simulink model "c00005M_harness"  (R2018a)
settings: Solver=ode3  StartTime=0.0  StopTime=10.0  RelTol=1e-3  EnableMultiTasking=on
undefined symbols (not defined in the file): b, DiscIntNeverNeededParam, J, K, L, PosMinimaW3, PosMinimaW4, R, sigbuilder_block
(part 19 of 75)

== system c00005M_harness/M080/Cyber ==
  note: Sensors
  note: Inputs For Window1
  note: Inputs for Window 2
  note: Inputs for window 3
  note: Inputs for window 4
  note: Users
  note: Users
  note: Sensors
  note: Users
  note: Sensors
  note: Users
  note: Sensors
  note: USERS
      | ---------------------------------
      | 0: None
      | 1: Ventana Arriba
      | 2: Ventana hasta arriba
      | 3: Ventana abajo
      | 4: Ventana hasta abajo
  note: 1: SUBE
      | 0: PARADO
      | -1 BAJA
  note: D = Driver (W1)
      | P1 = Passenger 1 (W2)
      | P2 = Passenger 2 (W3)
      | P3 = Passenger 3 (W4)
      | O = Obstacle
      | C = Control
      | Pri = Prioritizer
      | LD = LockDriver
      | PosW = PositionWindow
      | WL = WindowLogic
      | OW = ObstacleWindow
      | CWXC = ControlWindowXCentralized
      | S = Sensor
      | L = Lock
      | WPos = WindowPosition
      | M = Memory
      | InW = InputWindow
      | WIn = WindowInput
  PosW1 : Inport
  PosW2 : Inport  Port=2
  PosW3 : Inport  Port=3
  PosW4 : Inport  Port=4
  DW1 : Inport  Port=5
  DW3 : Inport  Port=6
  DW4 : Inport  Port=7
  P1W2 : Inport  Port=8
  P2W3 : Inport  Port=9
  P1W3 : Inport  Port=10
  P3W4 : Inport  Port=11
  OW1 : Inport  Port=12
  OW2 : Inport  Port=13
  OW3 : Inport  Port=14
  OW4 : Inport  Port=15
  LD : Inport  Port=16
  CW1C : Inport  Port=17
  CW2C : Inport  Port=18
  CW3C : Inport  Port=19
  CW4C : Inport  Port=20
  Pri : Subsystem
  Pri1 : Subsystem
  Pri3 : Subsystem
  Pri4 : Subsystem
  WL : Subsystem
  WL1 : Subsystem
  WL2 : Subsystem
  WL3 : Subsystem
  W1 : Outport
  W2 : Outport  Port=2
  W3 : Outport  Port=3
  W4 : Outport  Port=4
  wires:
  CW4C/1 -> Pri4/3(CW4C)
  CW3C/1 -> Pri1/4(CW3C)
  CW2C/1 -> Pri/2(CW2C)
  CW1C/1 -> Pri3/2(CW1C)
  Pri3/1(User) -> WL/2(User)
  WL3/1(WindowLogicOutput) -> W4/1
  WL2/1(WindowLogicOutput) -> W3/1
  Pri4/1(User) -> WL3/2(User)
  OW4/1 -> WL3/3(OW)
  PosW4/1 -> WL3/1(WPos)
  P3W4/1 -> Pri4/2(P)
  DW4/1 -> Pri4/1(D)
  P1W3/1 -> Pri1/3(P1)
  P2W3/1 -> Pri1/2(P)
  DW3/1 -> Pri1/1(D)
  OW3/1 -> WL2/3(OW)
  PosW3/1 -> WL2/1(WPos)
  Pri1/1(User) -> WL2/2(User)
  WL1/1(WindowLogicOutput) -> W2/1
  OW2/1 -> WL1/3(OW)
  PosW2/1 -> WL1/1(WPos)
  P1W2/1 -> Pri/1(P)
  Pri/1(User) -> WL1/2(User)
  WL/1(WindowLogicOutput) -> W1/1
  DW1/1 -> Pri3/1(D)
  OW1/1 -> WL/3(OW)
  PosW1/1 -> WL/1(WPos)
  LD/1 -> WL3/4(L)

== system c00005M_harness/M080/Physical ==
  InW1 : Inport
  InW2 : Inport  Port=2
  InW3 : Inport  Port=3
  InW4 : Inport  Port=4
  W : Subsystem
  W5 : Subsystem
  W6 : Subsystem
  W7 : Subsystem
  W1 : Outport
  W2 : Outport  Port=2
  W3 : Outport  Port=3
  W4 : Outport  Port=4
  wires:
  W7/1(WPos) -> W4/1
  W6/1(WPos) -> W3/1
  W5/1(WPos) -> W2/1
  W/1(WPos) -> W1/1
  InW4/1 -> W7/1(WIn)
  InW3/1 -> W6/1(WIn)
  InW2/1 -> W5/1(WIn)
  InW1/1 -> W/1(WIn)

== system c00005M_harness/M080/S1 ==
  PhyMeasure : Inport
  SensorOut : Outport
  wires:
  PhyMeasure/1 -> SensorOut/1

== system c00005M_harness/M080/S2 ==
  PhyMeasure : Inport
  SensorOut : Outport
  wires:
  PhyMeasure/1 -> SensorOut/1

== system c00005M_harness/M080/S3 ==
  PhyMeasure : Inport
  SensorOut : Outport
  wires:
  PhyMeasure/1 -> SensorOut/1

== system c00005M_harness/M080/S4 ==
  PhyMeasure : Inport
  SensorOut : Outport
  wires:
  PhyMeasure/1 -> SensorOut/1

== system c00005M_harness/M081/Cyber ==
  note: Sensors
  note: Inputs For Window1
  note: Inputs for Window 2
  note: Inputs for window 3
  note: Inputs for window 4
  note: Users
  note: Users
  note: Sensors
  note: Users
  note: Sensors
  note: Users
  note: Sensors
  note: USERS
      | ---------------------------------
      | 0: None
      | 1: Ventana Arriba
      | 2: Ventana hasta arriba
      | 3: Ventana abajo
      | 4: Ventana hasta abajo
  note: 1: SUBE
      | 0: PARADO
      | -1 BAJA
  note: D = Driver (W1)
      | P1 = Passenger 1 (W2)
      | P2 = Passenger 2 (W3)
      | P3 = Passenger 3 (W4)
      | O = Obstacle
      | C = Control
      | Pri = Prioritizer
      | LD = LockDriver
      | PosW = PositionWindow
      | WL = WindowLogic
      | OW = ObstacleWindow
      | CWXC = ControlWindowXCentralized
      | S = Sensor
      | L = Lock
      | WPos = WindowPosition
      | M = Memory
      | InW = InputWindow
      | WIn = WindowInput
  PosW1 : Inport
  PosW2 : Inport  Port=2
  PosW3 : Inport  Port=3
  PosW4 : Inport  Port=4
  DW1 : Inport  Port=5
  DW3 : Inport  Port=6
  DW4 : Inport  Port=7
  P1W2 : Inport  Port=8
  P2W3 : Inport  Port=9
  P1W3 : Inport  Port=10
  P3W4 : Inport  Port=11
  OW1 : Inport  Port=12
  OW2 : Inport  Port=13
  OW3 : Inport  Port=14
  OW4 : Inport  Port=15
  LD : Inport  Port=16
  CW1C : Inport  Port=17
  CW2C : Inport  Port=18
  CW3C : Inport  Port=19
  CW4C : Inport  Port=20
  Pri : Subsystem
  Pri1 : Subsystem
  Pri3 : Subsystem
  Pri4 : Subsystem
  WL : Subsystem
  WL1 : Subsystem
  WL2 : Subsystem
  WL3 : Subsystem
  W1 : Outport
  W2 : Outport  Port=2
  W3 : Outport  Port=3
  W4 : Outport  Port=4
  wires:
  CW4C/1 -> Pri4/3(CW4C)
  CW3C/1 -> Pri1/4(CW3C)
  CW2C/1 -> Pri/2(CW2C)
  CW1C/1 -> Pri3/2(CW1C)
  Pri3/1(User) -> WL/2(User)
  WL3/1(WindowLogicOutput) -> W4/1
  WL2/1(WindowLogicOutput) -> W3/1
  Pri4/1(User) -> WL3/2(User)
  OW4/1 -> WL3/3(OW)
  PosW4/1 -> WL3/1(WPos)
  P3W4/1 -> Pri4/2(P)
  DW4/1 -> Pri4/1(D)
  P1W3/1 -> Pri1/3(P1)
  P2W3/1 -> Pri1/2(P)
  DW3/1 -> Pri1/1(D)
  OW3/1 -> WL2/3(OW)
  PosW3/1 -> WL2/1(WPos)
  Pri1/1(User) -> WL2/2(User)
  WL1/1(WindowLogicOutput) -> W2/1
  OW2/1 -> WL1/3(OW)
  PosW2/1 -> WL1/1(WPos)
  P1W2/1 -> Pri/1(P)
  Pri/1(User) -> WL1/2(User)
  WL/1(WindowLogicOutput) -> W1/1
  DW1/1 -> Pri3/1(D)
  OW1/1 -> WL/3(OW)
  PosW1/1 -> WL/1(WPos)
  LD/1 -> WL3/4(L)

== system c00005M_harness/M081/Physical ==
  InW1 : Inport
  InW2 : Inport  Port=2
  InW3 : Inport  Port=3
  InW4 : Inport  Port=4
  W : Subsystem
  W5 : Subsystem
  W6 : Subsystem
  W7 : Subsystem
  W1 : Outport
  W2 : Outport  Port=2
  W3 : Outport  Port=3
  W4 : Outport  Port=4
  wires:
  W7/1(WPos) -> W4/1
  W6/1(WPos) -> W3/1
  W5/1(WPos) -> W2/1
  W/1(WPos) -> W1/1
  InW4/1 -> W7/1(WIn)
  InW3/1 -> W6/1(WIn)
  InW2/1 -> W5/1(WIn)
  InW1/1 -> W/1(WIn)

== system c00005M_harness/M081/S1 ==
  PhyMeasure : Inport
  SensorOut : Outport
  wires:
  PhyMeasure/1 -> SensorOut/1

== system c00005M_harness/M081/S2 ==
  PhyMeasure : Inport
  SensorOut : Outport
  wires:
  PhyMeasure/1 -> SensorOut/1

== system c00005M_harness/M081/S3 ==
  PhyMeasure : Inport
  SensorOut : Outport
  wires:
  PhyMeasure/1 -> SensorOut/1

== system c00005M_harness/M081/S4 ==
  PhyMeasure : Inport
  SensorOut : Outport
  wires:
  PhyMeasure/1 -> SensorOut/1

== system c00005M_harness/M082/Cyber ==
  note: Sensors
  note: Inputs For Window1
  note: Inputs for Window 2
  note: Inputs for window 3
  note: Inputs for window 4
  note: Users
  note: Users
  note: Sensors
  note: Users
  note: Sensors
  note: Users
  note: Sensors
  note: USERS
      | ---------------------------------
      | 0: None
      | 1: Ventana Arriba
      | 2: Ventana hasta arriba
      | 3: Ventana abajo
      | 4: Ventana hasta abajo
  note: 1: SUBE
      | 0: PARADO
      | -1 BAJA
  note: D = Driver (W1)
      | P1 = Passenger 1 (W2)
      | P2 = Passenger 2 (W3)
      | P3 = Passenger 3 (W4)
      | O = Obstacle
      | C = Control
      | Pri = Prioritizer
      | LD = LockDriver
      | PosW = PositionWindow
      | WL = WindowLogic
      | OW = ObstacleWindow
      | CWXC = ControlWindowXCentralized
      | S = Sensor
      | L = Lock
      | WPos = WindowPosition
      | M = Memory
      | InW = InputWindow
      | WIn = WindowInput
  PosW1 : Inport
  PosW2 : Inport  Port=2
  PosW3 : Inport  Port=3
  PosW4 : Inport  Port=4
  DW1 : Inport  Port=5
  DW3 : Inport  Port=6
  DW4 : Inport  Port=7
  P1W2 : Inport  Port=8
  P2W3 : Inport  Port=9
  P1W3 : Inport  Port=10
  P3W4 : Inport  Port=11
  OW1 : Inport  Port=12
  OW2 : Inport  Port=13
  OW3 : Inport  Port=14
  OW4 : Inport  Port=15
  LD : Inport  Port=16
  CW1C : Inport  Port=17
  CW2C : Inport  Port=18
  CW3C : Inport  Port=19
  CW4C : Inport  Port=20
  Pri : Subsystem
  Pri1 : Subsystem
  Pri3 : Subsystem
  Pri4 : Subsystem
  WL : Subsystem
  WL1 : Subsystem
  WL2 : Subsystem
  WL3 : Subsystem
  W1 : Outport
  W2 : Outport  Port=2
  W3 : Outport  Port=3
  W4 : Outport  Port=4
  wires:
  CW4C/1 -> Pri4/3(CW4C)
  CW3C/1 -> Pri1/4(CW3C)
  CW2C/1 -> Pri/2(CW2C)
  CW1C/1 -> Pri3/2(CW1C)
  Pri3/1(User) -> WL/2(User)
  WL3/1(WindowLogicOutput) -> W4/1
  WL2/1(WindowLogicOutput) -> W3/1
  Pri4/1(User) -> WL3/2(User)
  OW4/1 -> WL3/3(OW)
  PosW4/1 -> WL3/1(WPos)
  P3W4/1 -> Pri4/2(P)
  DW4/1 -> Pri4/1(D)
  P1W3/1 -> Pri1/3(P1)
  P2W3/1 -> Pri1/2(P)
  DW3/1 -> Pri1/1(D)
  OW3/1 -> WL2/3(OW)
  PosW3/1 -> WL2/1(WPos)
  Pri1/1(User) -> WL2/2(User)
  WL1/1(WindowLogicOutput) -> W2/1
  OW2/1 -> WL1/3(OW)
  PosW2/1 -> WL1/1(WPos)
  P1W2/1 -> Pri/1(P)
  Pri/1(User) -> WL1/2(User)
  WL/1(WindowLogicOutput) -> W1/1
  DW1/1 -> Pri3/1(D)
  OW1/1 -> WL/3(OW)
  PosW1/1 -> WL/1(WPos)
  LD/1 -> WL3/4(L)

== system c00005M_harness/M082/Physical ==
  InW1 : Inport
  InW2 : Inport  Port=2
  InW3 : Inport  Port=3
  InW4 : Inport  Port=4
  W : Subsystem
  W5 : Subsystem
  W6 : Subsystem
  W7 : Subsystem
  W1 : Outport
  W2 : Outport  Port=2
  W3 : Outport  Port=3
  W4 : Outport  Port=4
  wires:
  W7/1(WPos) -> W4/1
  W6/1(WPos) -> W3/1
  W5/1(WPos) -> W2/1
  W/1(WPos) -> W1/1
  InW4/1 -> W7/1(WIn)
  InW3/1 -> W6/1(WIn)
  InW2/1 -> W5/1(WIn)
  InW1/1 -> W/1(WIn)

== system c00005M_harness/M082/S1 ==
  PhyMeasure : Inport
  SensorOut : Outport
  wires:
  PhyMeasure/1 -> SensorOut/1

== system c00005M_harness/M082/S2 ==
  PhyMeasure : Inport
  SensorOut : Outport
  wires:
  PhyMeasure/1 -> SensorOut/1

== system c00005M_harness/M082/S3 ==
  PhyMeasure : Inport
  SensorOut : Outport
  wires:
  PhyMeasure/1 -> SensorOut/1

== system c00005M_harness/M082/S4 ==
  PhyMeasure : Inport
  SensorOut : Outport
  wires:
  PhyMeasure/1 -> SensorOut/1

== system c00005M_harness/M083/Cyber ==
  note: Sensors
  note: Inputs For Window1
  note: Inputs for Window 2
  note: Inputs for window 3
  note: Inputs for window 4
  note: Users
  note: Users
  note: Sensors
  note: Users
  note: Sensors
  note: Users
  note: Sensors
  note: USERS
      | ---------------------------------
      | 0: None
      | 1: Ventana Arriba
      | 2: Ventana hasta arriba
      | 3: Ventana abajo
      | 4: Ventana hasta abajo
  note: 1: SUBE
      | 0: PARADO
      | -1 BAJA
  note: D = Driver (W1)
      | P1 = Passenger 1 (W2)
      | P2 = Passenger 2 (W3)
      | P3 = Passenger 3 (W4)
      | O = Obstacle
      | C = Control
      | Pri = Prioritizer
      | LD = LockDriver
      | PosW = PositionWindow
      | WL = WindowLogic
      | OW = ObstacleWindow
      | CWXC = ControlWindowXCentralized
      | S = Sensor
      | L = Lock
      | WPos = WindowPosition
      | M = Memory
      | InW = InputWindow
      | WIn = WindowInput
  PosW1 : Inport
  PosW2 : Inport  Port=2
  PosW3 : Inport  Port=3
  PosW4 : Inport  Port=4
  DW1 : Inport  Port=5
  DW3 : Inport  Port=6
  DW4 : Inport  Port=7
  P1W2 : Inport  Port=8
  P2W3 : Inport  Port=9
  P1W3 : Inport  Port=10
  P3W4 : Inport  Port=11
  OW1 : Inport  Port=12
  OW2 : Inport  Port=13
  OW3 : Inport  Port=14
  OW4 : Inport  Port=15
  LD : Inport  Port=16
  CW1C : Inport  Port=17
  CW2C : Inport  Port=18
  CW3C : Inport  Port=19
  CW4C : Inport  Port=20
  Pri : Subsystem
  Pri1 : Subsystem
  Pri3 : Subsystem
  Pri4 : Subsystem
  WL : Subsystem
  WL1 : Subsystem
  WL2 : Subsystem
  WL3 : Subsystem
  W1 : Outport
  W2 : Outport  Port=2
  W3 : Outport  Port=3
  W4 : Outport  Port=4
  wires:
  CW4C/1 -> Pri4/3(CW4C)
  CW3C/1 -> Pri1/4(CW3C)
  CW2C/1 -> Pri/2(CW2C)
  CW1C/1 -> Pri3/2(CW1C)
  Pri3/1(User) -> WL/2(User)
  WL3/1(WindowLogicOutput) -> W4/1
  WL2/1(WindowLogicOutput) -> W3/1
  Pri4/1(User) -> WL3/2(User)
  OW4/1 -> WL3/3(OW)
  PosW4/1 -> WL3/1(WPos)
  P3W4/1 -> Pri4/2(P)
  DW4/1 -> Pri4/1(D)
  P1W3/1 -> Pri1/3(P1)
  P2W3/1 -> Pri1/2(P)
  DW3/1 -> Pri1/1(D)
  OW3/1 -> WL2/3(OW)
  PosW3/1 -> WL2/1(WPos)
  Pri1/1(User) -> WL2/2(User)
  WL1/1(WindowLogicOutput) -> W2/1
  OW2/1 -> WL1/3(OW)
  PosW2/1 -> WL1/1(WPos)
  P1W2/1 -> Pri/1(P)
  Pri/1(User) -> WL1/2(User)
  WL/1(WindowLogicOutput) -> W1/1
  DW1/1 -> Pri3/1(D)
  OW1/1 -> WL/3(OW)
  PosW1/1 -> WL/1(WPos)
  LD/1 -> WL3/4(L)

== system c00005M_harness/M083/Physical ==
  InW1 : Inport
  InW2 : Inport  Port=2
  InW3 : Inport  Port=3
  InW4 : Inport  Port=4
  W : Subsystem
  W5 : Subsystem
  W6 : Subsystem
  W7 : Subsystem
  W1 : Outport
  W2 : Outport  Port=2
  W3 : Outport  Port=3
  W4 : Outport  Port=4
  wires:
  W7/1(WPos) -> W4/1
  W6/1(WPos) -> W3/1
  W5/1(WPos) -> W2/1
  W/1(WPos) -> W1/1
  InW4/1 -> W7/1(WIn)
  InW3/1 -> W6/1(WIn)
  InW2/1 -> W5/1(WIn)
  InW1/1 -> W/1(WIn)

== system c00005M_harness/M083/S1 ==
  PhyMeasure : Inport
  SensorOut : Outport
  wires:
  PhyMeasure/1 -> SensorOut/1

== system c00005M_harness/M083/S2 ==
  PhyMeasure : Inport
  SensorOut : Outport
  wires:
  PhyMeasure/1 -> SensorOut/1

== system c00005M_harness/M083/S3 ==
  PhyMeasure : Inport
  SensorOut : Outport
  wires:
  PhyMeasure/1 -> SensorOut/1

== system c00005M_harness/M083/S4 ==
  PhyMeasure : Inport
  SensorOut : Outport
  wires:
  PhyMeasure/1 -> SensorOut/1

== system c00005M_harness/M084/Cyber ==
  note: Sensors
  note: Inputs For Window1
  note: Inputs for Window 2
  note: Inputs for window 3
  note: Inputs for window 4
  note: Users
  note: Users
  note: Sensors
  note: Users
  note: Sensors
  note: Users
  note: Sensors
  note: USERS
      | ---------------------------------
      | 0: None
      | 1: Ventana Arriba
      | 2: Ventana hasta arriba
      | 3: Ventana abajo
      | 4: Ventana hasta abajo
  note: 1: SUBE
      | 0: PARADO
      | -1 BAJA
  note: D = Driver (W1)
      | P1 = Passenger 1 (W2)
      | P2 = Passenger 2 (W3)
      | P3 = Passenger 3 (W4)
      | O = Obstacle
      | C = Control
      | Pri = Prioritizer
      | LD = LockDriver
      | PosW = PositionWindow
      | WL = WindowLogic
      | OW = ObstacleWindow
      | CWXC = ControlWindowXCentralized
      | S = Sensor
      | L = Lock
      | WPos = WindowPosition
      | M = Memory
      | InW = InputWindow
      | WIn = WindowInput
  PosW1 : Inport
  PosW2 : Inport  Port=2
  PosW3 : Inport  Port=3
  PosW4 : Inport  Port=4
  DW1 : Inport  Port=5
  DW3 : Inport  Port=6
  DW4 : Inport  Port=7
  P1W2 : Inport  Port=8
  P2W3 : Inport  Port=9
  P1W3 : Inport  Port=10
  P3W4 : Inport  Port=11
  OW1 : Inport  Port=12
  OW2 : Inport  Port=13
  OW3 : Inport  Port=14
  OW4 : Inport  Port=15
  LD : Inport  Port=16
  CW1C : Inport  Port=17
  CW2C : Inport  Port=18
  CW3C : Inport  Port=19
  CW4C : Inport  Port=20
  Pri : Subsystem
  Pri1 : Subsystem
  Pri3 : Subsystem
  Pri4 : Subsystem
  WL : Subsystem
  WL1 : Subsystem
  WL2 : Subsystem
  WL3 : Subsystem
  W1 : Outport
  W2 : Outport  Port=2
  W3 : Outport  Port=3
  W4 : Outport  Port=4
  wires:
  CW4C/1 -> Pri4/3(CW4C)
  CW3C/1 -> Pri1/4(CW3C)
  CW2C/1 -> Pri/2(CW2C)
  CW1C/1 -> Pri3/2(CW1C)
  Pri3/1(User) -> WL/2(User)
  WL3/1(WindowLogicOutput) -> W4/1
  WL2/1(WindowLogicOutput) -> W3/1
  Pri4/1(User) -> WL3/2(User)
  OW4/1 -> WL3/3(OW)
  PosW4/1 -> WL3/1(WPos)
  P3W4/1 -> Pri4/2(P)
  DW4/1 -> Pri4/1(D)
  P1W3/1 -> Pri1/3(P1)
  P2W3/1 -> Pri1/2(P)
  DW3/1 -> Pri1/1(D)
  OW3/1 -> WL2/3(OW)
  PosW3/1 -> WL2/1(WPos)
  Pri1/1(User) -> WL2/2(User)
  WL1/1(WindowLogicOutput) -> W2/1
  OW2/1 -> WL1/3(OW)
  PosW2/1 -> WL1/1(WPos)
  P1W2/1 -> Pri/1(P)
  Pri/1(User) -> WL1/2(User)
  WL/1(WindowLogicOutput) -> W1/1
  DW1/1 -> Pri3/1(D)
  OW1/1 -> WL/3(OW)
  PosW1/1 -> WL/1(WPos)
  LD/1 -> WL3/4(L)

== system c00005M_harness/M084/Physical ==
  InW1 : Inport
  InW2 : Inport  Port=2
  InW3 : Inport  Port=3
  InW4 : Inport  Port=4
  W : Subsystem
  W5 : Subsystem
  W6 : Subsystem
  W7 : Subsystem
  W1 : Outport
  W2 : Outport  Port=2
  W3 : Outport  Port=3
  W4 : Outport  Port=4
  wires:
  W7/1(WPos) -> W4/1
  W6/1(WPos) -> W3/1
  W5/1(WPos) -> W2/1
  W/1(WPos) -> W1/1
  InW4/1 -> W7/1(WIn)
  InW3/1 -> W6/1(WIn)
  InW2/1 -> W5/1(WIn)
  InW1/1 -> W/1(WIn)

== system c00005M_harness/M084/S1 ==
  PhyMeasure : Inport
  SensorOut : Outport
  wires:
  PhyMeasure/1 -> SensorOut/1

== system c00005M_harness/M084/S2 ==
  PhyMeasure : Inport
  SensorOut : Outport
  wires:
  PhyMeasure/1 -> SensorOut/1

== system c00005M_harness/M084/S3 ==
  PhyMeasure : Inport
  SensorOut : Outport
  wires:
  PhyMeasure/1 -> SensorOut/1

== system c00005M_harness/M084/S4 ==
  PhyMeasure : Inport
  SensorOut : Outport
  wires:
  PhyMeasure/1 -> SensorOut/1

== system c00005M_harness/M085/Cyber ==
  note: Sensors
  note: Inputs For Window1
  note: Inputs for Window 2
  note: Inputs for window 3
  note: Inputs for window 4
  note: Users
  note: Users
  note: Sensors
  note: Users
  note: Sensors
  note: Users
  note: Sensors
  note: USERS
      | ---------------------------------
      | 0: None
      | 1: Ventana Arriba
      | 2: Ventana hasta arriba
      | 3: Ventana abajo
      | 4: Ventana hasta abajo
  note: 1: SUBE
      | 0: PARADO
      | -1 BAJA
  note: D = Driver (W1)
      | P1 = Passenger 1 (W2)
      | P2 = Passenger 2 (W3)
      | P3 = Passenger 3 (W4)
      | O = Obstacle
      | C = Control
      | Pri = Prioritizer
      | LD = LockDriver
      | PosW = PositionWindow
      | WL = WindowLogic
      | OW = ObstacleWindow
      | CWXC = ControlWindowXCentralized
      | S = Sensor
      | L = Lock
      | WPos = WindowPosition
      | M = Memory
      | InW = InputWindow
      | WIn = WindowInput
  PosW1 : Inport
  PosW2 : Inport  Port=2
  PosW3 : Inport  Port=3
  PosW4 : Inport  Port=4
  DW1 : Inport  Port=5
  DW3 : Inport  Port=6
  DW4 : Inport  Port=7
  P1W2 : Inport  Port=8
  P2W3 : Inport  Port=9
  P1W3 : Inport  Port=10
  P3W4 : Inport  Port=11
  OW1 : Inport  Port=12
  OW2 : Inport  Port=13
  OW3 : Inport  Port=14
  OW4 : Inport  Port=15
  LD : Inport  Port=16
  CW1C : Inport  Port=17
  CW2C : Inport  Port=18
  CW3C : Inport  Port=19
  CW4C : Inport  Port=20
  Pri : Subsystem
  Pri1 : Subsystem
  Pri3 : Subsystem
  Pri4 : Subsystem
  WL : Subsystem
  WL1 : Subsystem
  WL2 : Subsystem
  WL3 : Subsystem
  W1 : Outport
  W2 : Outport  Port=2
  W3 : Outport  Port=3
  W4 : Outport  Port=4
  wires:
  CW4C/1 -> Pri4/3(CW4C)
  CW3C/1 -> Pri1/4(CW3C)
  CW2C/1 -> Pri/2(CW2C)
  CW1C/1 -> Pri3/2(CW1C)
  Pri3/1(User) -> WL/2(User)
  WL3/1(WindowLogicOutput) -> W4/1
  WL2/1(WindowLogicOutput) -> W3/1
  Pri4/1(User) -> WL3/2(User)
  OW4/1 -> WL3/3(OW)
  PosW4/1 -> WL3/1(WPos)
  P3W4/1 -> Pri4/2(P)
  DW4/1 -> Pri4/1(D)
  P1W3/1 -> Pri1/3(P1)
  P2W3/1 -> Pri1/2(P)
  DW3/1 -> Pri1/1(D)
  OW3/1 -> WL2/3(OW)
  PosW3/1 -> WL2/1(WPos)
  Pri1/1(User) -> WL2/2(User)
  WL1/1(WindowLogicOutput) -> W2/1
  OW2/1 -> WL1/3(OW)
  PosW2/1 -> WL1/1(WPos)
  P1W2/1 -> Pri/1(P)
  Pri/1(User) -> WL1/2(User)
  WL/1(WindowLogicOutput) -> W1/1
  DW1/1 -> Pri3/1(D)
  OW1/1 -> WL/3(OW)
  PosW1/1 -> WL/1(WPos)
  LD/1 -> WL3/4(L)

== system c00005M_harness/M085/Physical ==
  InW1 : Inport
  InW2 : Inport  Port=2
  InW3 : Inport  Port=3
  InW4 : Inport  Port=4
  W : Subsystem
  W5 : Subsystem
  W6 : Subsystem
  W7 : Subsystem
  W1 : Outport
  W2 : Outport  Port=2
  W3 : Outport  Port=3
  W4 : Outport  Port=4
  wires:
  W7/1(WPos) -> W4/1
  W6/1(WPos) -> W3/1
  W5/1(WPos) -> W2/1
  W/1(WPos) -> W1/1
  InW4/1 -> W7/1(WIn)
  InW3/1 -> W6/1(WIn)
  InW2/1 -> W5/1(WIn)
  InW1/1 -> W/1(WIn)

== system c00005M_harness/M085/S1 ==
  PhyMeasure : Inport
  SensorOut : Outport
  wires:
  PhyMeasure/1 -> SensorOut/1

== system c00005M_harness/M085/S2 ==
  PhyMeasure : Inport
  SensorOut : Outport
  wires:
  PhyMeasure/1 -> SensorOut/1

== system c00005M_harness/M085/S3 ==
  PhyMeasure : Inport
  SensorOut : Outport
  wires:
  PhyMeasure/1 -> SensorOut/1

== system c00005M_harness/M085/S4 ==
  PhyMeasure : Inport
  SensorOut : Outport
  wires:
  PhyMeasure/1 -> SensorOut/1

== system c00005M_harness/M086/Cyber ==
  note: Sensors
  note: Inputs For Window1
  note: Inputs for Window 2
  note: Inputs for window 3
  note: Inputs for window 4
  note: Users
  note: Users
  note: Sensors
  note: Users
  note: Sensors
  note: Users
  note: Sensors
  note: USERS
      | ---------------------------------
      | 0: None
      | 1: Ventana Arriba
      | 2: Ventana hasta arriba
      | 3: Ventana abajo
      | 4: Ventana hasta abajo
  note: 1: SUBE
      | 0: PARADO
      | -1 BAJA
  note: D = Driver (W1)
      | P1 = Passenger 1 (W2)
      | P2 = Passenger 2 (W3)
      | P3 = Passenger 3 (W4)
      | O = Obstacle
      | C = Control
      | Pri = Prioritizer
      | LD = LockDriver
      | PosW = PositionWindow
      | WL = WindowLogic
      | OW = ObstacleWindow
      | CWXC = ControlWindowXCentralized
      | S = Sensor
      | L = Lock
      | WPos = WindowPosition
      | M = Memory
      | InW = InputWindow
      | WIn = WindowInput
  PosW1 : Inport
  PosW2 : Inport  Port=2
  PosW3 : Inport  Port=3
  PosW4 : Inport  Port=4
  DW1 : Inport  Port=5
  DW3 : Inport  Port=6
  DW4 : Inport  Port=7
  P1W2 : Inport  Port=8
  P2W3 : Inport  Port=9
  P1W3 : Inport  Port=10
  P3W4 : Inport  Port=11
  OW1 : Inport  Port=12
  OW2 : Inport  Port=13
  OW3 : Inport  Port=14
  OW4 : Inport  Port=15
  LD : Inport  Port=16
  CW1C : Inport  Port=17
  CW2C : Inport  Port=18
  CW3C : Inport  Port=19
  CW4C : Inport  Port=20
  Pri : Subsystem
  Pri1 : Subsystem
  Pri3 : Subsystem
  Pri4 : Subsystem
  WL : Subsystem
  WL1 : Subsystem
  WL2 : Subsystem
  WL3 : Subsystem
  W1 : Outport
  W2 : Outport  Port=2
  W3 : Outport  Port=3
  W4 : Outport  Port=4
  wires:
  CW4C/1 -> Pri4/3(CW4C)
  CW3C/1 -> Pri1/4(CW3C)
  CW2C/1 -> Pri/2(CW2C)
  CW1C/1 -> Pri3/2(CW1C)
  Pri3/1(User) -> WL/2(User)
  WL3/1(WindowLogicOutput) -> W4/1
  WL2/1(WindowLogicOutput) -> W3/1
  Pri4/1(User) -> WL3/2(User)
  OW4/1 -> WL3/3(OW)
  PosW4/1 -> WL3/1(WPos)
  P3W4/1 -> Pri4/2(P)
  DW4/1 -> Pri4/1(D)
  P1W3/1 -> Pri1/3(P1)
  P2W3/1 -> Pri1/2(P)
  DW3/1 -> Pri1/1(D)
  OW3/1 -> WL2/3(OW)
  PosW3/1 -> WL2/1(WPos)
  Pri1/1(User) -> WL2/2(User)
  WL1/1(WindowLogicOutput) -> W2/1
  OW2/1 -> WL1/3(OW)
  PosW2/1 -> WL1/1(WPos)
  P1W2/1 -> Pri/1(P)
  Pri/1(User) -> WL1/2(User)
  WL/1(WindowLogicOutput) -> W1/1
  DW1/1 -> Pri3/1(D)
  OW1/1 -> WL/3(OW)
  PosW1/1 -> WL/1(WPos)
  LD/1 -> WL3/4(L)

== system c00005M_harness/M086/Physical ==
  InW1 : Inport
  InW2 : Inport  Port=2
  InW3 : Inport  Port=3
  InW4 : Inport  Port=4
  W : Subsystem
  W5 : Subsystem
  W6 : Subsystem
  W7 : Subsystem
  W1 : Outport
  W2 : Outport  Port=2
  W3 : Outport  Port=3
  W4 : Outport  Port=4
  wires:
  W7/1(WPos) -> W4/1
  W6/1(WPos) -> W3/1
  W5/1(WPos) -> W2/1
  W/1(WPos) -> W1/1
  InW4/1 -> W7/1(WIn)
  InW3/1 -> W6/1(WIn)
  InW2/1 -> W5/1(WIn)
  InW1/1 -> W/1(WIn)

== system c00005M_harness/M086/S1 ==
  PhyMeasure : Inport
  SensorOut : Outport
  wires:
  PhyMeasure/1 -> SensorOut/1

== system c00005M_harness/M086/S2 ==
  PhyMeasure : Inport
  SensorOut : Outport
  wires:
  PhyMeasure/1 -> SensorOut/1

== system c00005M_harness/M086/S3 ==
  PhyMeasure : Inport
  SensorOut : Outport
  wires:
  PhyMeasure/1 -> SensorOut/1

== system c00005M_harness/M086/S4 ==
  PhyMeasure : Inport
  SensorOut : Outport
  wires:
  PhyMeasure/1 -> SensorOut/1

== system c00005M_harness/M087/Cyber ==
  note: Sensors
  note: Inputs For Window1
  note: Inputs for Window 2
  note: Inputs for window 3
  note: Inputs for window 4
  note: Users
  note: Users
  note: Sensors
  note: Users
  note: Sensors
  note: Users
  note: Sensors
  note: USERS
      | ---------------------------------
      | 0: None
      | 1: Ventana Arriba
      | 2: Ventana hasta arriba
      | 3: Ventana abajo
      | 4: Ventana hasta abajo
  note: 1: SUBE
      | 0: PARADO
      | -1 BAJA
  note: D = Driver (W1)
      | P1 = Passenger 1 (W2)
      | P2 = Passenger 2 (W3)
      | P3 = Passenger 3 (W4)
      | O = Obstacle
      | C = Control
      | Pri = Prioritizer
      | LD = LockDriver
      | PosW = PositionWindow
      | WL = WindowLogic
      | OW = ObstacleWindow
      | CWXC = ControlWindowXCentralized
      | S = Sensor
      | L = Lock
      | WPos = WindowPosition
      | M = Memory
      | InW = InputWindow
      | WIn = WindowInput
  PosW1 : Inport
  PosW2 : Inport  Port=2
  PosW3 : Inport  Port=3
  PosW4 : Inport  Port=4
  DW1 : Inport  Port=5
  DW3 : Inport  Port=6
  DW4 : Inport  Port=7
  P1W2 : Inport  Port=8
  P2W3 : Inport  Port=9
  P1W3 : Inport  Port=10
  P3W4 : Inport  Port=11
  OW1 : Inport  Port=12
  OW2 : Inport  Port=13
  OW3 : Inport  Port=14
  OW4 : Inport  Port=15
  LD : Inport  Port=16
  CW1C : Inport  Port=17
  CW2C : Inport  Port=18
  CW3C : Inport  Port=19
  CW4C : Inport  Port=20
  Pri : Subsystem
  Pri1 : Subsystem
  Pri3 : Subsystem
  Pri4 : Subsystem
  WL : Subsystem
  WL1 : Subsystem
  WL2 : Subsystem
  WL3 : Subsystem
  W1 : Outport
  W2 : Outport  Port=2
  W3 : Outport  Port=3
  W4 : Outport  Port=4
  wires:
  CW4C/1 -> Pri4/3(CW4C)
  CW3C/1 -> Pri1/4(CW3C)
  CW2C/1 -> Pri/2(CW2C)
  CW1C/1 -> Pri3/2(CW1C)
  Pri3/1(User) -> WL/2(User)
  WL3/1(WindowLogicOutput) -> W4/1
  WL2/1(WindowLogicOutput) -> W3/1
  Pri4/1(User) -> WL3/2(User)
  OW4/1 -> WL3/3(OW)
  PosW4/1 -> WL3/1(WPos)
  P3W4/1 -> Pri4/2(P)
  DW4/1 -> Pri4/1(D)
  P1W3/1 -> Pri1/3(P1)
  P2W3/1 -> Pri1/2(P)
  DW3/1 -> Pri1/1(D)
  OW3/1 -> WL2/3(OW)
  PosW3/1 -> WL2/1(WPos)
  Pri1/1(User) -> WL2/2(User)
  WL1/1(WindowLogicOutput) -> W2/1
  OW2/1 -> WL1/3(OW)
  PosW2/1 -> WL1/1(WPos)
  P1W2/1 -> Pri/1(P)
  Pri/1(User) -> WL1/2(User)
  WL/1(WindowLogicOutput) -> W1/1
  DW1/1 -> Pri3/1(D)
  OW1/1 -> WL/3(OW)
  PosW1/1 -> WL/1(WPos)
  LD/1 -> WL3/4(L)

== system c00005M_harness/M087/Physical ==
  InW1 : Inport
  InW2 : Inport  Port=2
  InW3 : Inport  Port=3
  InW4 : Inport  Port=4
  W : Subsystem
  W5 : Subsystem
  W6 : Subsystem
  W7 : Subsystem
  W1 : Outport
  W2 : Outport  Port=2
  W3 : Outport  Port=3
  W4 : Outport  Port=4
  wires:
  W7/1(WPos) -> W4/1
  W6/1(WPos) -> W3/1
  W5/1(WPos) -> W2/1
  W/1(WPos) -> W1/1
  InW4/1 -> W7/1(WIn)
  InW3/1 -> W6/1(WIn)
  InW2/1 -> W5/1(WIn)
  InW1/1 -> W/1(WIn)

== system c00005M_harness/M087/S1 ==
  PhyMeasure : Inport
  SensorOut : Outport
  wires:
  PhyMeasure/1 -> SensorOut/1

== system c00005M_harness/M087/S2 ==
  PhyMeasure : Inport
  SensorOut : Outport
  wires:
  PhyMeasure/1 -> SensorOut/1

== system c00005M_harness/M087/S3 ==
  PhyMeasure : Inport
  SensorOut : Outport
  wires:
  PhyMeasure/1 -> SensorOut/1

== system c00005M_harness/M087/S4 ==
  PhyMeasure : Inport
  SensorOut : Outport
  wires:
  PhyMeasure/1 -> SensorOut/1

== system c00005M_harness/M088/Cyber ==
  note: Sensors
  note: Inputs For Window1
  note: Inputs for Window 2
  note: Inputs for window 3
  note: Inputs for window 4
  note: Users
  note: Users
  note: Sensors
  note: Users
  note: Sensors
  note: Users
  note: Sensors
  note: USERS
      | ---------------------------------
      | 0: None
      | 1: Ventana Arriba
      | 2: Ventana hasta arriba
      | 3: Ventana abajo
      | 4: Ventana hasta abajo
  note: 1: SUBE
      | 0: PARADO
      | -1 BAJA
  note: D = Driver (W1)
      | P1 = Passenger 1 (W2)
      | P2 = Passenger 2 (W3)
      | P3 = Passenger 3 (W4)
      | O = Obstacle
      | C = Control
      | Pri = Prioritizer
      | LD = LockDriver
      | PosW = PositionWindow
      | WL = WindowLogic
      | OW = ObstacleWindow
      | CWXC = ControlWindowXCentralized
      | S = Sensor
      | L = Lock
      | WPos = WindowPosition
      | M = Memory
      | InW = InputWindow
      | WIn = WindowInput
  PosW1 : Inport
  PosW2 : Inport  Port=2
  PosW3 : Inport  Port=3
  PosW4 : Inport  Port=4
  DW1 : Inport  Port=5
  DW3 : Inport  Port=6
  DW4 : Inport  Port=7
  P1W2 : Inport  Port=8
  P2W3 : Inport  Port=9
  P1W3 : Inport  Port=10
  P3W4 : Inport  Port=11
  OW1 : Inport  Port=12
  OW2 : Inport  Port=13
  OW3 : Inport  Port=14
  OW4 : Inport  Port=15
  LD : Inport  Port=16
  CW1C : Inport  Port=17
  CW2C : Inport  Port=18
  CW3C : Inport  Port=19
  CW4C : Inport  Port=20
  Pri : Subsystem
  Pri1 : Subsystem
  Pri3 : Subsystem
  Pri4 : Subsystem
  WL : Subsystem
  WL1 : Subsystem
  WL2 : Subsystem
  WL3 : Subsystem
  W1 : Outport
  W2 : Outport  Port=2
  W3 : Outport  Port=3
  W4 : Outport  Port=4
  wires:
  CW4C/1 -> Pri4/3(CW4C)
  CW3C/1 -> Pri1/4(CW3C)
  CW2C/1 -> Pri/2(CW2C)
  CW1C/1 -> Pri3/2(CW1C)
  Pri3/1(User) -> WL/2(User)
  WL3/1(WindowLogicOutput) -> W4/1
  WL2/1(WindowLogicOutput) -> W3/1
  Pri4/1(User) -> WL3/2(User)
  OW4/1 -> WL3/3(OW)
  PosW4/1 -> WL3/1(WPos)
  P3W4/1 -> Pri4/2(P)
  DW4/1 -> Pri4/1(D)
  P1W3/1 -> Pri1/3(P1)
  P2W3/1 -> Pri1/2(P)
  DW3/1 -> Pri1/1(D)
  OW3/1 -> WL2/3(OW)
  PosW3/1 -> WL2/1(WPos)
  Pri1/1(User) -> WL2/2(User)
  WL1/1(WindowLogicOutput) -> W2/1
  OW2/1 -> WL1/3(OW)
  PosW2/1 -> WL1/1(WPos)
  P1W2/1 -> Pri/1(P)
  Pri/1(User) -> WL1/2(User)
  WL/1(WindowLogicOutput) -> W1/1
  DW1/1 -> Pri3/1(D)
  OW1/1 -> WL/3(OW)
  PosW1/1 -> WL/1(WPos)
  LD/1 -> WL3/4(L)

== system c00005M_harness/M088/Physical ==
  InW1 : Inport
  InW2 : Inport  Port=2
  InW3 : Inport  Port=3
  InW4 : Inport  Port=4
  W : Subsystem
  W5 : Subsystem
  W6 : Subsystem
  W7 : Subsystem
  W1 : Outport
  W2 : Outport  Port=2
  W3 : Outport  Port=3
  W4 : Outport  Port=4
  wires:
  W7/1(WPos) -> W4/1
  W6/1(WPos) -> W3/1
  W5/1(WPos) -> W2/1
  W/1(WPos) -> W1/1
  InW4/1 -> W7/1(WIn)
  InW3/1 -> W6/1(WIn)
  InW2/1 -> W5/1(WIn)
  InW1/1 -> W/1(WIn)

== system c00005M_harness/M088/S1 ==
  PhyMeasure : Inport
  SensorOut : Outport
  wires:
  PhyMeasure/1 -> SensorOut/1

== system c00005M_harness/M088/S2 ==
  PhyMeasure : Inport
  SensorOut : Outport
  wires:
  PhyMeasure/1 -> SensorOut/1

== system c00005M_harness/M088/S3 ==
  PhyMeasure : Inport
  SensorOut : Outport
  wires:
  PhyMeasure/1 -> SensorOut/1

== system c00005M_harness/M088/S4 ==
  PhyMeasure : Inport
  SensorOut : Outport
  wires:
  PhyMeasure/1 -> SensorOut/1

== system c00005M_harness/M089/Cyber ==
  note: Sensors
  note: Inputs For Window1
  note: Inputs for Window 2
  note: Inputs for window 3
  note: Inputs for window 4
  note: Users
  note: Users
  note: Sensors
  note: Users
  note: Sensors
  note: Users
  note: Sensors
  note: USERS
      | ---------------------------------
      | 0: None
      | 1: Ventana Arriba
      | 2: Ventana hasta arriba
      | 3: Ventana abajo
      | 4: Ventana hasta abajo
  note: 1: SUBE
      | 0: PARADO
      | -1 BAJA
  note: D = Driver (W1)
      | P1 = Passenger 1 (W2)
      | P2 = Passenger 2 (W3)
      | P3 = Passenger 3 (W4)
      | O = Obstacle
      | C = Control
      | Pri = Prioritizer
      | LD = LockDriver
      | PosW = PositionWindow
      | WL = WindowLogic
      | OW = ObstacleWindow
      | CWXC = ControlWindowXCentralized
      | S = Sensor
      | L = Lock
      | WPos = WindowPosition
      | M = Memory
      | InW = InputWindow
      | WIn = WindowInput
  PosW1 : Inport
  PosW2 : Inport  Port=2
  PosW3 : Inport  Port=3
  PosW4 : Inport  Port=4
  DW1 : Inport  Port=5
  DW3 : Inport  Port=6
  DW4 : Inport  Port=7
  P1W2 : Inport  Port=8
  P2W3 : Inport  Port=9
  P1W3 : Inport  Port=10
  P3W4 : Inport  Port=11
  OW1 : Inport  Port=12
  OW2 : Inport  Port=13
  OW3 : Inport  Port=14
  OW4 : Inport  Port=15
  LD : Inport  Port=16
  CW1C : Inport  Port=17
  CW2C : Inport  Port=18
  CW3C : Inport  Port=19
  CW4C : Inport  Port=20
  Pri : Subsystem
  Pri1 : Subsystem
  Pri3 : Subsystem
  Pri4 : Subsystem
  WL : Subsystem
  WL1 : Subsystem
  WL2 : Subsystem
  WL3 : Subsystem
  W1 : Outport
  W2 : Outport  Port=2
  W3 : Outport  Port=3
  W4 : Outport  Port=4
  wires:
  CW4C/1 -> Pri4/3(CW4C)
  CW3C/1 -> Pri1/4(CW3C)
  CW2C/1 -> Pri/2(CW2C)
  CW1C/1 -> Pri3/2(CW1C)
  Pri3/1(User) -> WL/2(User)
  WL3/1(WindowLogicOutput) -> W4/1
  WL2/1(WindowLogicOutput) -> W3/1
  Pri4/1(User) -> WL3/2(User)
  OW4/1 -> WL3/3(OW)
  PosW4/1 -> WL3/1(WPos)
  P3W4/1 -> Pri4/2(P)
  DW4/1 -> Pri4/1(D)
  P1W3/1 -> Pri1/3(P1)
  P2W3/1 -> Pri1/2(P)
  DW3/1 -> Pri1/1(D)
  OW3/1 -> WL2/3(OW)
  PosW3/1 -> WL2/1(WPos)
  Pri1/1(User) -> WL2/2(User)
  WL1/1(WindowLogicOutput) -> W2/1
  OW2/1 -> WL1/3(OW)
  PosW2/1 -> WL1/1(WPos)
  P1W2/1 -> Pri/1(P)
  Pri/1(User) -> WL1/2(User)
  WL/1(WindowLogicOutput) -> W1/1
  DW1/1 -> Pri3/1(D)
  OW1/1 -> WL/3(OW)
  PosW1/1 -> WL/1(WPos)
  LD/1 -> WL3/4(L)

== system c00005M_harness/M089/Physical ==
  InW1 : Inport
  InW2 : Inport  Port=2
  InW3 : Inport  Port=3
  InW4 : Inport  Port=4
  W : Subsystem
  W5 : Subsystem
  W6 : Subsystem
  W7 : Subsystem
  W1 : Outport
  W2 : Outport  Port=2
  W3 : Outport  Port=3
  W4 : Outport  Port=4
  wires:
  W7/1(WPos) -> W4/1
  W6/1(WPos) -> W3/1
  W5/1(WPos) -> W2/1
  W/1(WPos) -> W1/1
  InW4/1 -> W7/1(WIn)
  InW3/1 -> W6/1(WIn)
  InW2/1 -> W5/1(WIn)
  InW1/1 -> W/1(WIn)

== system c00005M_harness/M089/S1 ==
  PhyMeasure : Inport
  SensorOut : Outport
  wires:
  PhyMeasure/1 -> SensorOut/1

== system c00005M_harness/M089/S2 ==
  PhyMeasure : Inport
  SensorOut : Outport
  wires:
  PhyMeasure/1 -> SensorOut/1

== system c00005M_harness/M089/S3 ==
  PhyMeasure : Inport
  SensorOut : Outport
  wires:
  PhyMeasure/1 -> SensorOut/1

== system c00005M_harness/M089/S4 ==
  PhyMeasure : Inport
  SensorOut : Outport
  wires:
  PhyMeasure/1 -> SensorOut/1

== system c00005M_harness/M090/Cyber ==
  note: Sensors
  note: Inputs For Window1
  note: Inputs for Window 2
  note: Inputs for window 3
  note: Inputs for window 4
  note: Users
  note: Users
  note: Sensors
  note: Users
  note: Sensors
  note: Users
  note: Sensors
  note: USERS
      | ---------------------------------
      | 0: None
      | 1: Ventana Arriba
      | 2: Ventana hasta arriba
      | 3: Ventana abajo
      | 4: Ventana hasta abajo
  note: 1: SUBE
      | 0: PARADO
      | -1 BAJA
  note: D = Driver (W1)
      | P1 = Passenger 1 (W2)
      | P2 = Passenger 2 (W3)
      | P3 = Passenger 3 (W4)
      | O = Obstacle
      | C = Control
      | Pri = Prioritizer
      | LD = LockDriver
      | PosW = PositionWindow
      | WL = WindowLogic
      | OW = ObstacleWindow
      | CWXC = ControlWindowXCentralized
      | S = Sensor
      | L = Lock
      | WPos = WindowPosition
      | M = Memory
      | InW = InputWindow
      | WIn = WindowInput
  PosW1 : Inport
  PosW2 : Inport  Port=2
  PosW3 : Inport  Port=3
  PosW4 : Inport  Port=4
  DW1 : Inport  Port=5
  DW3 : Inport  Port=6
  DW4 : Inport  Port=7
  P1W2 : Inport  Port=8
  P2W3 : Inport  Port=9
  P1W3 : Inport  Port=10
  P3W4 : Inport  Port=11
  OW1 : Inport  Port=12
  OW2 : Inport  Port=13
  OW3 : Inport  Port=14
  OW4 : Inport  Port=15
  LD : Inport  Port=16
  CW1C : Inport  Port=17
  CW2C : Inport  Port=18
  CW3C : Inport  Port=19
  CW4C : Inport  Port=20
  Pri : Subsystem
  Pri1 : Subsystem
  Pri3 : Subsystem
  Pri4 : Subsystem
  WL : Subsystem
  WL1 : Subsystem
  WL2 : Subsystem
  WL3 : Subsystem
  W1 : Outport
  W2 : Outport  Port=2
  W3 : Outport  Port=3
  W4 : Outport  Port=4
  wires:
  CW4C/1 -> Pri4/3(CW4C)
  CW3C/1 -> Pri1/4(CW3C)
  CW2C/1 -> Pri/2(CW2C)
  CW1C/1 -> Pri3/2(CW1C)
  Pri3/1(User) -> WL/2(User)
  WL3/1(WindowLogicOutput) -> W4/1
  WL2/1(WindowLogicOutput) -> W3/1
  Pri4/1(User) -> WL3/2(User)
  OW4/1 -> WL3/3(OW)
  PosW4/1 -> WL3/1(WPos)
  P3W4/1 -> Pri4/2(P)
  DW4/1 -> Pri4/1(D)
  P1W3/1 -> Pri1/3(P1)
  P2W3/1 -> Pri1/2(P)
  DW3/1 -> Pri1/1(D)
  OW3/1 -> WL2/3(OW)
  PosW3/1 -> WL2/1(WPos)
  Pri1/1(User) -> WL2/2(User)
  WL1/1(WindowLogicOutput) -> W2/1
  OW2/1 -> WL1/3(OW)
  PosW2/1 -> WL1/1(WPos)
  P1W2/1 -> Pri/1(P)
  Pri/1(User) -> WL1/2(User)
  WL/1(WindowLogicOutput) -> W1/1
  DW1/1 -> Pri3/1(D)
  OW1/1 -> WL/3(OW)
  PosW1/1 -> WL/1(WPos)
  LD/1 -> WL3/4(L)

== system c00005M_harness/M090/Physical ==
  InW1 : Inport
  InW2 : Inport  Port=2
  InW3 : Inport  Port=3
  InW4 : Inport  Port=4
  W : Subsystem
  W5 : Subsystem
  W6 : Subsystem
  W7 : Subsystem
  W1 : Outport
  W2 : Outport  Port=2
  W3 : Outport  Port=3
  W4 : Outport  Port=4
  wires:
  W7/1(WPos) -> W4/1
  W6/1(WPos) -> W3/1
  W5/1(WPos) -> W2/1
  W/1(WPos) -> W1/1
  InW4/1 -> W7/1(WIn)
  InW3/1 -> W6/1(WIn)
  InW2/1 -> W5/1(WIn)
  InW1/1 -> W/1(WIn)

== system c00005M_harness/M090/S1 ==
  PhyMeasure : Inport
  SensorOut : Outport
  wires:
  PhyMeasure/1 -> SensorOut/1

== system c00005M_harness/M090/S2 ==
  PhyMeasure : Inport
  SensorOut : Outport
  wires:
  PhyMeasure/1 -> SensorOut/1

== system c00005M_harness/M090/S3 ==
  PhyMeasure : Inport
  SensorOut : Outport
  wires:
  PhyMeasure/1 -> SensorOut/1

== system c00005M_harness/M090/S4 ==
  PhyMeasure : Inport
  SensorOut : Outport
  wires:
  PhyMeasure/1 -> SensorOut/1

== system c00005M_harness/M091/Cyber ==
  note: Sensors
  note: Inputs For Window1
  note: Inputs for Window 2
  note: Inputs for window 3
  note: Inputs for window 4
  note: Users
  note: Users
  note: Sensors
  note: Users
  note: Sensors
  note: Users
  note: Sensors
  note: USERS
      | ---------------------------------
      | 0: None
      | 1: Ventana Arriba
      | 2: Ventana hasta arriba
      | 3: Ventana abajo
      | 4: Ventana hasta abajo
  note: 1: SUBE
      | 0: PARADO
      | -1 BAJA
  note: D = Driver (W1)
      | P1 = Passenger 1 (W2)
      | P2 = Passenger 2 (W3)
      | P3 = Passenger 3 (W4)
      | O = Obstacle
      | C = Control
      | Pri = Prioritizer
      | LD = LockDriver
      | PosW = PositionWindow
      | WL = WindowLogic
      | OW = ObstacleWindow
      | CWXC = ControlWindowXCentralized
      | S = Sensor
      | L = Lock
      | WPos = WindowPosition
      | M = Memory
      | InW = InputWindow
      | WIn = WindowInput
  PosW1 : Inport
  PosW2 : Inport  Port=2
  PosW3 : Inport  Port=3
  PosW4 : Inport  Port=4
  DW1 : Inport  Port=5
  DW3 : Inport  Port=6
  DW4 : Inport  Port=7
  P1W2 : Inport  Port=8
  P2W3 : Inport  Port=9
  P1W3 : Inport  Port=10
  P3W4 : Inport  Port=11
  OW1 : Inport  Port=12
  OW2 : Inport  Port=13
  OW3 : Inport  Port=14
  OW4 : Inport  Port=15
  LD : Inport  Port=16
  CW1C : Inport  Port=17
  CW2C : Inport  Port=18
  CW3C : Inport  Port=19
  CW4C : Inport  Port=20
  Pri : Subsystem
  Pri1 : Subsystem
  Pri3 : Subsystem
  Pri4 : Subsystem
  WL : Subsystem
  WL1 : Subsystem
  WL2 : Subsystem
  WL3 : Subsystem
  W1 : Outport
  W2 : Outport  Port=2
  W3 : Outport  Port=3
  W4 : Outport  Port=4
  wires:
  CW4C/1 -> Pri4/3(CW4C)
  CW3C/1 -> Pri1/4(CW3C)
  CW2C/1 -> Pri/2(CW2C)
  CW1C/1 -> Pri3/2(CW1C)
  Pri3/1(User) -> WL/2(User)
  WL3/1(WindowLogicOutput) -> W4/1
  WL2/1(WindowLogicOutput) -> W3/1
  Pri4/1(User) -> WL3/2(User)
  OW4/1 -> WL3/3(OW)
  PosW4/1 -> WL3/1(WPos)
  P3W4/1 -> Pri4/2(P)
  DW4/1 -> Pri4/1(D)
  P1W3/1 -> Pri1/3(P1)
  P2W3/1 -> Pri1/2(P)
  DW3/1 -> Pri1/1(D)
  OW3/1 -> WL2/3(OW)
  PosW3/1 -> WL2/1(WPos)
  Pri1/1(User) -> WL2/2(User)
  WL1/1(WindowLogicOutput) -> W2/1
  OW2/1 -> WL1/3(OW)
  PosW2/1 -> WL1/1(WPos)
  P1W2/1 -> Pri/1(P)
  Pri/1(User) -> WL1/2(User)
  WL/1(WindowLogicOutput) -> W1/1
  DW1/1 -> Pri3/1(D)
  OW1/1 -> WL/3(OW)
  PosW1/1 -> WL/1(WPos)
  LD/1 -> WL3/4(L)

== system c00005M_harness/M091/Physical ==
  InW1 : Inport
  InW2 : Inport  Port=2
  InW3 : Inport  Port=3
  InW4 : Inport  Port=4
  W : Subsystem
  W5 : Subsystem
  W6 : Subsystem
  W7 : Subsystem
  W1 : Outport
  W2 : Outport  Port=2
  W3 : Outport  Port=3
  W4 : Outport  Port=4
  wires:
  W7/1(WPos) -> W4/1
  W6/1(WPos) -> W3/1
  W5/1(WPos) -> W2/1
  W/1(WPos) -> W1/1
  InW4/1 -> W7/1(WIn)
  InW3/1 -> W6/1(WIn)
  InW2/1 -> W5/1(WIn)
  InW1/1 -> W/1(WIn)

== system c00005M_harness/M091/S1 ==
  PhyMeasure : Inport
  SensorOut : Outport
  wires:
  PhyMeasure/1 -> SensorOut/1

== system c00005M_harness/M091/S2 ==
  PhyMeasure : Inport
  SensorOut : Outport
  wires:
  PhyMeasure/1 -> SensorOut/1

== system c00005M_harness/M091/S3 ==
  PhyMeasure : Inport
  SensorOut : Outport
  wires:
  PhyMeasure/1 -> SensorOut/1

== system c00005M_harness/M091/S4 ==
  PhyMeasure : Inport
  SensorOut : Outport
  wires:
  PhyMeasure/1 -> SensorOut/1

== system c00005M_harness/M092/Cyber ==
  note: Sensors
  note: Inputs For Window1
  note: Inputs for Window 2
  note: Inputs for window 3
  note: Inputs for window 4
  note: Users
  note: Users
  note: Sensors
  note: Users
  note: Sensors
  note: Users
  note: Sensors
  note: USERS
      | ---------------------------------
      | 0: None
      | 1: Ventana Arriba
      | 2: Ventana hasta arriba
      | 3: Ventana abajo
      | 4: Ventana hasta abajo
  note: 1: SUBE
      | 0: PARADO
      | -1 BAJA
  note: D = Driver (W1)
      | P1 = Passenger 1 (W2)
      | P2 = Passenger 2 (W3)
      | P3 = Passenger 3 (W4)
      | O = Obstacle
      | C = Control
      | Pri = Prioritizer
      | LD = LockDriver
      | PosW = PositionWindow
      | WL = WindowLogic
      | OW = ObstacleWindow
      | CWXC = ControlWindowXCentralized
      | S = Sensor
      | L = Lock
      | WPos = WindowPosition
      | M = Memory
      | InW = InputWindow
      | WIn = WindowInput
  PosW1 : Inport
  PosW2 : Inport  Port=2
  PosW3 : Inport  Port=3
  PosW4 : Inport  Port=4
  DW1 : Inport  Port=5
  DW3 : Inport  Port=6
  DW4 : Inport  Port=7
  P1W2 : Inport  Port=8
  P2W3 : Inport  Port=9
  P1W3 : Inport  Port=10
  P3W4 : Inport  Port=11
  OW1 : Inport  Port=12
  OW2 : Inport  Port=13
  OW3 : Inport  Port=14
  OW4 : Inport  Port=15
  LD : Inport  Port=16
  CW1C : Inport  Port=17
  CW2C : Inport  Port=18
  CW3C : Inport  Port=19
  CW4C : Inport  Port=20
  Pri : Subsystem
  Pri1 : Subsystem
  Pri3 : Subsystem
  Pri4 : Subsystem
  WL : Subsystem
  WL1 : Subsystem
  WL2 : Subsystem
  WL3 : Subsystem
  W1 : Outport
  W2 : Outport  Port=2
  W3 : Outport  Port=3
  W4 : Outport  Port=4
  wires:
  CW4C/1 -> Pri4/3(CW4C)
  CW3C/1 -> Pri1/4(CW3C)
  CW2C/1 -> Pri/2(CW2C)
  CW1C/1 -> Pri3/2(CW1C)
  Pri3/1(User) -> WL/2(User)
  WL3/1(WindowLogicOutput) -> W4/1
  WL2/1(WindowLogicOutput) -> W3/1
  Pri4/1(User) -> WL3/2(User)
  OW4/1 -> WL3/3(OW)
  PosW4/1 -> WL3/1(WPos)
  P3W4/1 -> Pri4/2(P)
  DW4/1 -> Pri4/1(D)
  P1W3/1 -> Pri1/3(P1)
  P2W3/1 -> Pri1/2(P)
  DW3/1 -> Pri1/1(D)
  OW3/1 -> WL2/3(OW)
  PosW3/1 -> WL2/1(WPos)
  Pri1/1(User) -> WL2/2(User)
  WL1/1(WindowLogicOutput) -> W2/1
  OW2/1 -> WL1/3(OW)
  PosW2/1 -> WL1/1(WPos)
  P1W2/1 -> Pri/1(P)
  Pri/1(User) -> WL1/2(User)
  WL/1(WindowLogicOutput) -> W1/1
  DW1/1 -> Pri3/1(D)
  OW1/1 -> WL/3(OW)
  PosW1/1 -> WL/1(WPos)
  LD/1 -> WL3/4(L)

== system c00005M_harness/M092/Physical ==
  InW1 : Inport
  InW2 : Inport  Port=2
  InW3 : Inport  Port=3
  InW4 : Inport  Port=4
  W : Subsystem
  W5 : Subsystem
  W6 : Subsystem
  W7 : Subsystem
  W1 : Outport
  W2 : Outport  Port=2
  W3 : Outport  Port=3
  W4 : Outport  Port=4
  wires:
  W7/1(WPos) -> W4/1
  W6/1(WPos) -> W3/1
  W5/1(WPos) -> W2/1
  W/1(WPos) -> W1/1
  InW4/1 -> W7/1(WIn)
  InW3/1 -> W6/1(WIn)
  InW2/1 -> W5/1(WIn)
  InW1/1 -> W/1(WIn)

== system c00005M_harness/M092/S1 ==
  PhyMeasure : Inport
  SensorOut : Outport
  wires:
  PhyMeasure/1 -> SensorOut/1

== system c00005M_harness/M092/S2 ==
  PhyMeasure : Inport
  SensorOut : Outport
  wires:
  PhyMeasure/1 -> SensorOut/1

== system c00005M_harness/M092/S3 ==
  PhyMeasure : Inport
  SensorOut : Outport
  wires:
  PhyMeasure/1 -> SensorOut/1

== system c00005M_harness/M092/S4 ==
  PhyMeasure : Inport
  SensorOut : Outport
  wires:
  PhyMeasure/1 -> SensorOut/1

== system c00005M_harness/M093/Cyber ==
  note: Sensors
  note: Inputs For Window1
  note: Inputs for Window 2
  note: Inputs for window 3
  note: Inputs for window 4
  note: Users
  note: Users
  note: Sensors
  note: Users
  note: Sensors
  note: Users
  note: Sensors
  note: USERS
      | ---------------------------------
      | 0: None
      | 1: Ventana Arriba
      | 2: Ventana hasta arriba
      | 3: Ventana abajo
      | 4: Ventana hasta abajo
  note: 1: SUBE
      | 0: PARADO
      | -1 BAJA
  note: D = Driver (W1)
      | P1 = Passenger 1 (W2)
      | P2 = Passenger 2 (W3)
      | P3 = Passenger 3 (W4)
      | O = Obstacle
      | C = Control
      | Pri = Prioritizer
      | LD = LockDriver
      | PosW = PositionWindow
      | WL = WindowLogic
      | OW = ObstacleWindow
      | CWXC = ControlWindowXCentralized
      | S = Sensor
      | L = Lock
      | WPos = WindowPosition
      | M = Memory
      | InW = InputWindow
      | WIn = WindowInput
  PosW1 : Inport
  PosW2 : Inport  Port=2
  PosW3 : Inport  Port=3
  PosW4 : Inport  Port=4
  DW1 : Inport  Port=5
  DW3 : Inport  Port=6
  DW4 : Inport  Port=7
  P1W2 : Inport  Port=8
  P2W3 : Inport  Port=9
  P1W3 : Inport  Port=10
  P3W4 : Inport  Port=11
  OW1 : Inport  Port=12
  OW2 : Inport  Port=13
  OW3 : Inport  Port=14
  OW4 : Inport  Port=15
  LD : Inport  Port=16
  CW1C : Inport  Port=17
  CW2C : Inport  Port=18
  CW3C : Inport  Port=19
  CW4C : Inport  Port=20
  Pri : Subsystem
  Pri1 : Subsystem
  Pri3 : Subsystem
  Pri4 : Subsystem
  WL : Subsystem
  WL1 : Subsystem
  WL2 : Subsystem
  WL3 : Subsystem
  W1 : Outport
  W2 : Outport  Port=2
  W3 : Outport  Port=3
  W4 : Outport  Port=4
  wires:
  CW4C/1 -> Pri4/3(CW4C)
  CW3C/1 -> Pri1/4(CW3C)
  CW2C/1 -> Pri/2(CW2C)
  CW1C/1 -> Pri3/2(CW1C)
  Pri3/1(User) -> WL/2(User)
  WL3/1(WindowLogicOutput) -> W4/1
  WL2/1(WindowLogicOutput) -> W3/1
  Pri4/1(User) -> WL3/2(User)
  OW4/1 -> WL3/3(OW)
  PosW4/1 -> WL3/1(WPos)
  P3W4/1 -> Pri4/2(P)
  DW4/1 -> Pri4/1(D)
  P1W3/1 -> Pri1/3(P1)
  P2W3/1 -> Pri1/2(P)
  DW3/1 -> Pri1/1(D)
  OW3/1 -> WL2/3(OW)
  PosW3/1 -> WL2/1(WPos)
  Pri1/1(User) -> WL2/2(User)
  WL1/1(WindowLogicOutput) -> W2/1
  OW2/1 -> WL1/3(OW)
  PosW2/1 -> WL1/1(WPos)
  P1W2/1 -> Pri/1(P)
  Pri/1(User) -> WL1/2(User)
  WL/1(WindowLogicOutput) -> W1/1
  DW1/1 -> Pri3/1(D)
  OW1/1 -> WL/3(OW)
  PosW1/1 -> WL/1(WPos)
  LD/1 -> WL3/4(L)

== system c00005M_harness/M093/Physical ==
  InW1 : Inport
  InW2 : Inport  Port=2
  InW3 : Inport  Port=3
  InW4 : Inport  Port=4
  W : Subsystem
  W5 : Subsystem
  W6 : Subsystem
  W7 : Subsystem
  W1 : Outport
  W2 : Outport  Port=2
  W3 : Outport  Port=3
  W4 : Outport  Port=4
  wires:
  W7/1(WPos) -> W4/1
  W6/1(WPos) -> W3/1
  W5/1(WPos) -> W2/1
  W/1(WPos) -> W1/1
  InW4/1 -> W7/1(WIn)
  InW3/1 -> W6/1(WIn)
  InW2/1 -> W5/1(WIn)
  InW1/1 -> W/1(WIn)

== system c00005M_harness/M093/S1 ==
  PhyMeasure : Inport
  SensorOut : Outport
  wires:
  PhyMeasure/1 -> SensorOut/1

== system c00005M_harness/M093/S2 ==
  PhyMeasure : Inport
  SensorOut : Outport
  wires:
  PhyMeasure/1 -> SensorOut/1

== system c00005M_harness/M093/S3 ==
  PhyMeasure : Inport
  SensorOut : Outport
  wires:
  PhyMeasure/1 -> SensorOut/1

== system c00005M_harness/M093/S4 ==
  PhyMeasure : Inport
  SensorOut : Outport
  wires:
  PhyMeasure/1 -> SensorOut/1

== system c00005M_harness/M094/Cyber ==
  note: Sensors
  note: Inputs For Window1
  note: Inputs for Window 2
  note: Inputs for window 3
  note: Inputs for window 4
  note: Users
  note: Users
  note: Sensors
  note: Users
  note: Sensors
  note: Users
  note: Sensors
  note: USERS
      | ---------------------------------
      | 0: None
      | 1: Ventana Arriba
      | 2: Ventana hasta arriba
      | 3: Ventana abajo
      | 4: Ventana hasta abajo
  note: 1: SUBE
      | 0: PARADO
      | -1 BAJA
  note: D = Driver (W1)
      | P1 = Passenger 1 (W2)
      | P2 = Passenger 2 (W3)
      | P3 = Passenger 3 (W4)
      | O = Obstacle
      | C = Control
      | Pri = Prioritizer
      | LD = LockDriver
      | PosW = PositionWindow
      | WL = WindowLogic
      | OW = ObstacleWindow
      | CWXC = ControlWindowXCentralized
      | S = Sensor
      | L = Lock
      | WPos = WindowPosition
      | M = Memory
      | InW = InputWindow
      | WIn = WindowInput
  PosW1 : Inport
  PosW2 : Inport  Port=2
  PosW3 : Inport  Port=3
  PosW4 : Inport  Port=4
  DW1 : Inport  Port=5
  DW3 : Inport  Port=6
  DW4 : Inport  Port=7
  P1W2 : Inport  Port=8
  P2W3 : Inport  Port=9
  P1W3 : Inport  Port=10
  P3W4 : Inport  Port=11
  OW1 : Inport  Port=12
  OW2 : Inport  Port=13
  OW3 : Inport  Port=14
  OW4 : Inport  Port=15
  LD : Inport  Port=16
  CW1C : Inport  Port=17
  CW2C : Inport  Port=18
  CW3C : Inport  Port=19
  CW4C : Inport  Port=20
  Pri : Subsystem
  Pri1 : Subsystem
  Pri3 : Subsystem
  Pri4 : Subsystem
  WL : Subsystem
  WL1 : Subsystem
  WL2 : Subsystem
  WL3 : Subsystem
  W1 : Outport
  W2 : Outport  Port=2
  W3 : Outport  Port=3
  W4 : Outport  Port=4
  wires:
  CW4C/1 -> Pri4/3(CW4C)
  CW3C/1 -> Pri1/4(CW3C)
  CW2C/1 -> Pri/2(CW2C)
  CW1C/1 -> Pri3/2(CW1C)
  Pri3/1(User) -> WL/2(User)
  WL3/1(WindowLogicOutput) -> W4/1
  WL2/1(WindowLogicOutput) -> W3/1
  Pri4/1(User) -> WL3/2(User)
  OW4/1 -> WL3/3(OW)
  PosW4/1 -> WL3/1(WPos)
  P3W4/1 -> Pri4/2(P)
  DW4/1 -> Pri4/1(D)
  P1W3/1 -> Pri1/3(P1)
  P2W3/1 -> Pri1/2(P)
  DW3/1 -> Pri1/1(D)
  OW3/1 -> WL2/3(OW)
  PosW3/1 -> WL2/1(WPos)
  Pri1/1(User) -> WL2/2(User)
  WL1/1(WindowLogicOutput) -> W2/1
  OW2/1 -> WL1/3(OW)
  PosW2/1 -> WL1/1(WPos)
  P1W2/1 -> Pri/1(P)
  Pri/1(User) -> WL1/2(User)
  WL/1(WindowLogicOutput) -> W1/1
  DW1/1 -> Pri3/1(D)
  OW1/1 -> WL/3(OW)
  PosW1/1 -> WL/1(WPos)
  LD/1 -> WL3/4(L)

== system c00005M_harness/M094/Physical ==
  InW1 : Inport
  InW2 : Inport  Port=2
  InW3 : Inport  Port=3
  InW4 : Inport  Port=4
  W : Subsystem
  W5 : Subsystem
  W6 : Subsystem
  W7 : Subsystem
  W1 : Outport
  W2 : Outport  Port=2
  W3 : Outport  Port=3
  W4 : Outport  Port=4
  wires:
  W7/1(WPos) -> W4/1
  W6/1(WPos) -> W3/1
  W5/1(WPos) -> W2/1
  W/1(WPos) -> W1/1
  InW4/1 -> W7/1(WIn)
  InW3/1 -> W6/1(WIn)
  InW2/1 -> W5/1(WIn)
  InW1/1 -> W/1(WIn)

== system c00005M_harness/M094/S1 ==
  PhyMeasure : Inport
  SensorOut : Outport
  wires:
  PhyMeasure/1 -> SensorOut/1

== system c00005M_harness/M094/S2 ==
  PhyMeasure : Inport
  SensorOut : Outport
  wires:
  PhyMeasure/1 -> SensorOut/1

== system c00005M_harness/M094/S3 ==
  PhyMeasure : Inport
  SensorOut : Outport
  wires:
  PhyMeasure/1 -> SensorOut/1

== system c00005M_harness/M094/S4 ==
  PhyMeasure : Inport
  SensorOut : Outport
  wires:
  PhyMeasure/1 -> SensorOut/1

== system c00005M_harness/M095/Cyber ==
  note: Sensors
  note: Inputs For Window1
  note: Inputs for Window 2
  note: Inputs for window 3
  note: Inputs for window 4
  note: Users
  note: Users
  note: Sensors
  note: Users
  note: Sensors
  note: Users
  note: Sensors
  note: USERS
      | ---------------------------------
      | 0: None
      | 1: Ventana Arriba
      | 2: Ventana hasta arriba
      | 3: Ventana abajo
      | 4: Ventana hasta abajo
  note: 1: SUBE
      | 0: PARADO
      | -1 BAJA
  note: D = Driver (W1)
      | P1 = Passenger 1 (W2)
      | P2 = Passenger 2 (W3)
      | P3 = Passenger 3 (W4)
      | O = Obstacle
      | C = Control
      | Pri = Prioritizer
      | LD = LockDriver
      | PosW = PositionWindow
      | WL = WindowLogic
      | OW = ObstacleWindow
      | CWXC = ControlWindowXCentralized
      | S = Sensor
      | L = Lock
      | WPos = WindowPosition
      | M = Memory
      | InW = InputWindow
      | WIn = WindowInput
  PosW1 : Inport
  PosW2 : Inport  Port=2
  PosW3 : Inport  Port=3
  PosW4 : Inport  Port=4
  DW1 : Inport  Port=5
  DW3 : Inport  Port=6
  DW4 : Inport  Port=7
  P1W2 : Inport  Port=8
  P2W3 : Inport  Port=9
  P1W3 : Inport  Port=10
  P3W4 : Inport  Port=11
  OW1 : Inport  Port=12
  OW2 : Inport  Port=13
  OW3 : Inport  Port=14
  OW4 : Inport  Port=15
  LD : Inport  Port=16
  CW1C : Inport  Port=17
  CW2C : Inport  Port=18
  CW3C : Inport  Port=19
  CW4C : Inport  Port=20
  Pri : Subsystem
  Pri1 : Subsystem
  Pri3 : Subsystem
  Pri4 : Subsystem
  WL : Subsystem
  WL1 : Subsystem
  WL2 : Subsystem
  WL3 : Subsystem
  W1 : Outport
  W2 : Outport  Port=2
  W3 : Outport  Port=3
  W4 : Outport  Port=4
  wires:
  CW4C/1 -> Pri4/3(CW4C)
  CW3C/1 -> Pri1/4(CW3C)
  CW2C/1 -> Pri/2(CW2C)
  CW1C/1 -> Pri3/2(CW1C)
  Pri3/1(User) -> WL/2(User)
  WL3/1(WindowLogicOutput) -> W4/1
  WL2/1(WindowLogicOutput) -> W3/1
  Pri4/1(User) -> WL3/2(User)
  OW4/1 -> WL3/3(OW)
  PosW4/1 -> WL3/1(WPos)
  P3W4/1 -> Pri4/2(P)
  DW4/1 -> Pri4/1(D)
  P1W3/1 -> Pri1/3(P1)
  P2W3/1 -> Pri1/2(P)
  DW3/1 -> Pri1/1(D)
  OW3/1 -> WL2/3(OW)
  PosW3/1 -> WL2/1(WPos)
  Pri1/1(User) -> WL2/2(User)
  WL1/1(WindowLogicOutput) -> W2/1
  OW2/1 -> WL1/3(OW)
  PosW2/1 -> WL1/1(WPos)
  P1W2/1 -> Pri/1(P)
  Pri/1(User) -> WL1/2(User)
  WL/1(WindowLogicOutput) -> W1/1
  DW1/1 -> Pri3/1(D)
  OW1/1 -> WL/3(OW)
  PosW1/1 -> WL/1(WPos)
  LD/1 -> WL3/4(L)
